simulink model "modelGreenHydrogenPlant"  (R2025a)
settings: Solver=ode1  StartTime=0.0  StopTime=exe.tsim  FixedStep=exe.tstep  RelTol=1e-3
undefined symbols (not defined in the file): Chosen_Strategy, DiscIntNeverNeededParam, ELY, ESS, exe, fb, Grid, grid, Ib2, Kc, kd, Ki_cc_cp, Ki_Inertia_Less, Kp_cc_cp, kp_GFo, Kp_Inertia_Less, PV, R, Rload, Sb, SCLR, t_ELY_on, Theta_Vvsc0, Time_Step, Va0, Vb0, Vb1, Vb2, Vc0, Vm0, VSC01_id0, Vvsc0, wb, Zb
libraries: spsSeriesRLCBranchLib x18, spsCurrentMeasurementLib x17, spsVoltageMeasurementLib x15, Control_Lib x13, spsRMSLib x8, simulink x8, spsabctodq0Lib x7, spsThreePhaseBreakerLib x5, spsPowerdq0InstantaneousLib x4, spsGroundLib x3, spsUniversalBridgeLib x3, spsControlledVoltageSourceLib x3
(part 1 of 3)
settings Model: Creator=kauchr  LastModifiedBy=kauchr
settings OptimizationCC: ReuseModelBlockBuffer=off
settings RTWCC: GPUComputeCapability=3.5

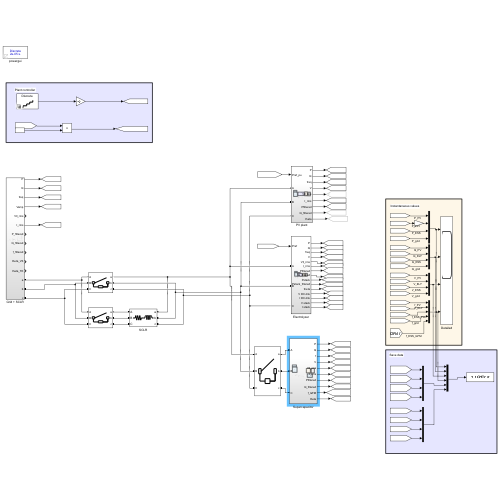
[thumbnail: Simulink's stored preview of the top-level diagram]
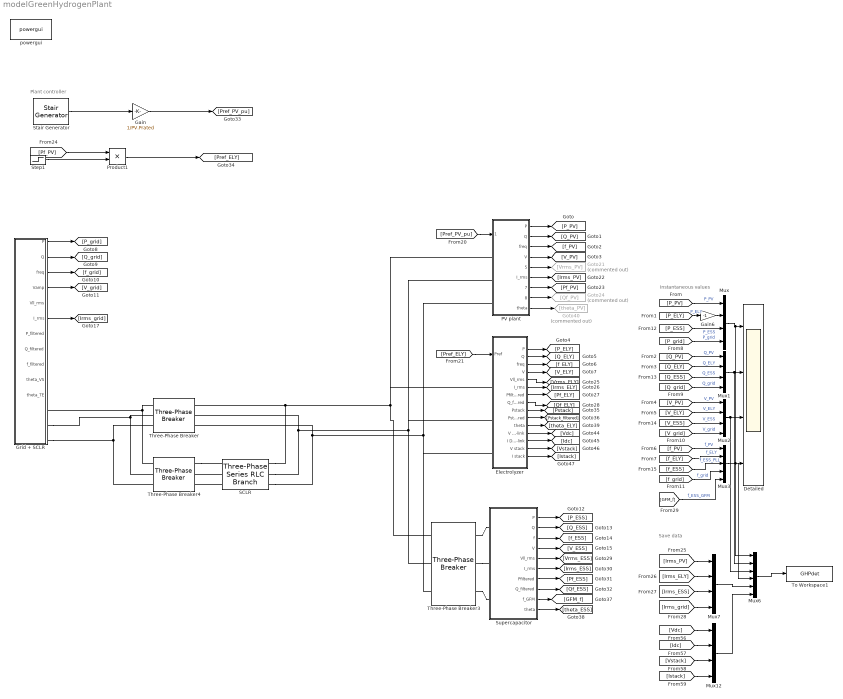
== system modelGreenHydrogenPlant ==
  note: Plant controller
  note: Instantaneous values
  note: Save data
  Detailed : Scope  NumInputPorts=4
      settings: Title=Active power  ActiveDisplayYMinimum=-22041.76945  ActiveDisplayYMaximum=60401.48573  YLabel=Active power (W)
  Electrolyzer : Subsystem
  Gain : Gain  Gain=1/PV.Prated
  Gain6 : Gain  Gain=-1
  Goto21 : Goto  Commented=on  GotoTag=Vrms_PV
  Goto24 : Goto  Commented=on  GotoTag=Qf_PV
  Goto40 : Goto  Commented=on  GotoTag=theta_PV
  Grid + SCLR : Subsystem
  Mux{,1..2,7,12} (5 alike) : Mux
  Mux3 : Mux  Inputs=5
  Mux6 : Mux  Inputs=6
  PV plant : Subsystem
  Product1 : Product
  SCLR : spsThreePhaseSeriesRLCBranchLib/Three-Phase Series RLC Branch  LConnTagsString=A|B|C  RConnTagsString=A|B|C  BranchType=RL  Resistance=SCLR.R  Inductance=SCLR.L  Capacitance=1e-6  Measurements=None
  Stair Generator : eeStairGenerator/Stair Generator  LabelModeActiveChoice=Discrete  TimeInput=setP_t  AmplitudeInput=setP_P  SampleTime=exe.tstep  RepeatPattern=off  OutDataTypeStr=double
      settings: LibrarySourceBlock=ee_sl_lib/General Control/Stair Generator
  Step1 : Step  Time=t_ELY_on  SampleTime=0
  Supercapacitor : Subsystem
  Three-Phase Breaker : spsThreePhaseBreakerLib/Three-Phase Breaker  InitialState=open  SwitchA=on  SwitchB=on  SwitchC=on  SwitchTimes="[Grid.CB.on  Grid.CB.off]"  External=off  BreakerResistance=0.01  SnubberResistance=1e6  SnubberCapacitance=inf  Measurements=None
  Three-Phase Breaker3 : spsThreePhaseBreakerLib/Three-Phase Breaker  InitialState=open  SwitchA=on  SwitchB=on  SwitchC=on  SwitchTimes="[ESS.CB.on  ESS.CB.off]"  External=off  BreakerResistance=1e-6  SnubberResistance=1e6  SnubberCapacitance=inf  Measurements=None
  Three-Phase Breaker4 : spsThreePhaseBreakerLib/Three-Phase Breaker  InitialState=open  SwitchA=on  SwitchB=on  SwitchC=on  SwitchTimes="[SCLR.CB.on  SCLR.CB.off]"  External=off  BreakerResistance=0.01  SnubberResistance=1e6  SnubberCapacitance=inf  Measurements=None
  To Workspace1 : ToWorkspace  VariableName=GHPdet  SaveFormat=Timeseries  SampleTime=1e-3
  powergui : sps_lib/powergui  Priority=1  SimulationMode=Discrete  SampleTime=exe.tstep  frequency=60  Iterations=50  frequencyindice=0  Pbase=100e6  ErrMax=1e-4  UnitsV=kV  UnitsW=MW  buscounter=0  FunctionMessages=off  echomessages=off  EnableUseOfTLC=off  CurrentSourceSwitches=off  DisableSnubberDevices=off  DisableRonSwitches=off  DisableVfSwitches=off  DisplayEquations=off  AutomaticDiscreteSolvers=off  SolverType=Tustin/Backward Euler (TBE)  Interpol=off  ExternalGateDelay=off  methode=off  Ts=100  x0status=blocks  SPID=on  SwTol=0  HookPort=off  NonlinearTolerance=1e-4  nMaxIteration=100  ContinueOnMaxIteration=off  RestoreLinks=warning  ResistiveCurrentMeasurement=off  Frange=[0:2:500]  Ylog=off  Xlog=on  ShowGrid=off  save=off  variable=ZData  structure=0  ZoomFFT=off  StartTime=0.0  cycles=1  DisplayStyle=1  fundamental=60  FreqAxis=off  MaxFrequency=1000  frequencyindicesteady=1  RmsSteady=1  display=off
  wires:
  PV plant/1(P) -> [P_PV]
  PV plant/2(Q) -> [Q_PV]
  PV plant/3(freq) -> [f_PV]
  PV plant/4(V) -> [V_PV]
  Electrolyzer/4(V) -> [V_ELY]
  Electrolyzer/1(P) -> [P_ELY]
  Electrolyzer/2(Q) -> [Q_ELY]
  Electrolyzer/3(freq) -> [f_ELY]
  [P_PV] -> Mux/1  "P_PV"
  [P_ELY] -> Gain6/1  "P_ELY"
  [Q_ELY] -> Mux1/2  "Q_ELY"
  [Q_PV] -> Mux1/1  "Q_PV"
  [V_PV] -> Mux2/1  "V_PV"
  [V_ELY] -> Mux2/2  "V_ELY"
  [f_ELY] -> Mux3/2  "f_ELY"
  [f_PV] -> Mux3/1  "f_PV"
  Mux/1 -> Mux6/1, Detailed/1
  Mux1/1 -> Mux6/2, Detailed/2
  Mux2/1 -> Mux6/3, Detailed/3
  Mux3/1 -> Mux6/4, Detailed/4
  Supercapacitor/1(P) -> [P_ESS]
  Supercapacitor/2(Q) -> [Q_ESS]
  Supercapacitor/3(f) -> [f_ESS]
  Supercapacitor/4(V) -> [V_ESS]
  [P_ESS] -> Mux/3  "P_ESS"
  [P_grid] -> Mux/4  "P_grid"
  [Q_ESS] -> Mux1/3  "Q_ESS"
  [Q_grid] -> Mux1/4  "Q_grid"
  [V_grid] -> Mux2/4  "V_grid"
  [V_ESS] -> Mux2/3  "V_ESS"
  [f_ESS] -> Mux3/3  "f_ESS_PLL"
  [f_grid] -> Mux3/4  "f_grid"
  PV plant/6(I_rms) -> [Irms_PV]
  PV plant/5(Vll_rms) -> Goto21/1
  PV plant/7(Pfiltered) -> [Pf_PV]
  PV plant/8(Q_filtered) -> Goto24/1
  Electrolyzer/5(Vll_rms) -> [Vrms_ELY]
  Electrolyzer/6(I_rms) -> [Irms_ELY]
  Electrolyzer/7(Pfiltered) -> [Pf_ELY]
  Electrolyzer/8(Q_filtered) -> [Qf_ELY]
  Supercapacitor/5(Vll_rms) -> [Vrms_ESS]
  Supercapacitor/6(I_rms) -> [Irms_ESS]
  Supercapacitor/7(Pfiltered) -> [Pf_ESS]
  Supercapacitor/8(Q_filtered) -> [Qf_ESS]
  Grid + SCLR/1(P) -> [P_grid]
  Grid + SCLR/2(Q) -> [Q_grid]
  Grid + SCLR/3(freq) -> [f_grid]
  Grid + SCLR/4(Vamp) -> [V_grid]
  Grid + SCLR/6(I_rms) -> [Irms_grid]
  [Pref_PV_pu] -> PV plant/1(Pref_pu)
  [Pref_ELY] -> Electrolyzer/1(Pref)
  Gain/1 -> [Pref_PV_pu]
  Step1/1 -> Product1/2
  Stair Generator/1 -> Gain/1
  Gain6/1 -> Mux/2
  Electrolyzer/9(Pstack) -> [Pstack]
  Electrolyzer/10(Pstack_filtered) -> [Pstack_filtered]
  [Irms_grid] -> Mux7/4
  Mux7/1 -> Mux6/5
  [Irms_PV] -> Mux7/1
  [Irms_ELY] -> Mux7/2
  Mux6/1 -> To Workspace1/1
  [Irms_ESS] -> Mux7/3
  Supercapacitor/9(f_GFM) -> [GFM_f]
  [GFM_f] -> Mux3/5  "f_ESS_GFM"
  Supercapacitor/10(theta) -> [theta_ESS]
  Electrolyzer/11(theta) -> [theta_ELY]
  PV plant/9(theta) -> Goto40/1
  [Pf_PV] -> Product1/1
  Electrolyzer/12(V DC-link) -> [Vdc]
  Electrolyzer/13(I DC-link) -> [Idc]
  Electrolyzer/14(V stack) -> [Vstack]
  Electrolyzer/15(I stack) -> [Istack]
  Mux12/1 -> Mux6/6
  [Vdc] -> Mux12/1
  [Idc] -> Mux12/2
  [Vstack] -> Mux12/3
  [Istack] -> Mux12/4
  Product1/1 -> [Pref_ELY]
  connections:
  Three-Phase Breaker/LConn1 -- Three-Phase Breaker4/LConn1 -- Grid + SCLR/RConn1
  Grid + SCLR/RConn2 -- Three-Phase Breaker/LConn2 -- Three-Phase Breaker4/LConn2
  Grid + SCLR/RConn3 -- Three-Phase Breaker/LConn3 -- Three-Phase Breaker4/LConn3
  Three-Phase Breaker4/RConn1 -- SCLR/LConn1
  SCLR/LConn3 -- Three-Phase Breaker4/RConn3
  SCLR/LConn2 -- Three-Phase Breaker4/RConn2
  Three-Phase Breaker3/RConn1 -- Supercapacitor/LConn1
  Three-Phase Breaker3/RConn2 -- Supercapacitor/LConn2
  Three-Phase Breaker3/RConn3 -- Supercapacitor/LConn3
  SCLR/RConn3 -- Three-Phase Breaker3/LConn3 -- Electrolyzer/LConn3 -- PV plant/LConn3 -- Three-Phase Breaker/RConn3
  SCLR/RConn2 -- Three-Phase Breaker/RConn2 -- Three-Phase Breaker3/LConn2 -- PV plant/LConn2 -- Electrolyzer/LConn2
  Three-Phase Breaker3/LConn1 -- PV plant/LConn1 -- Electrolyzer/LConn1 -- SCLR/RConn1 -- Three-Phase Breaker/RConn1

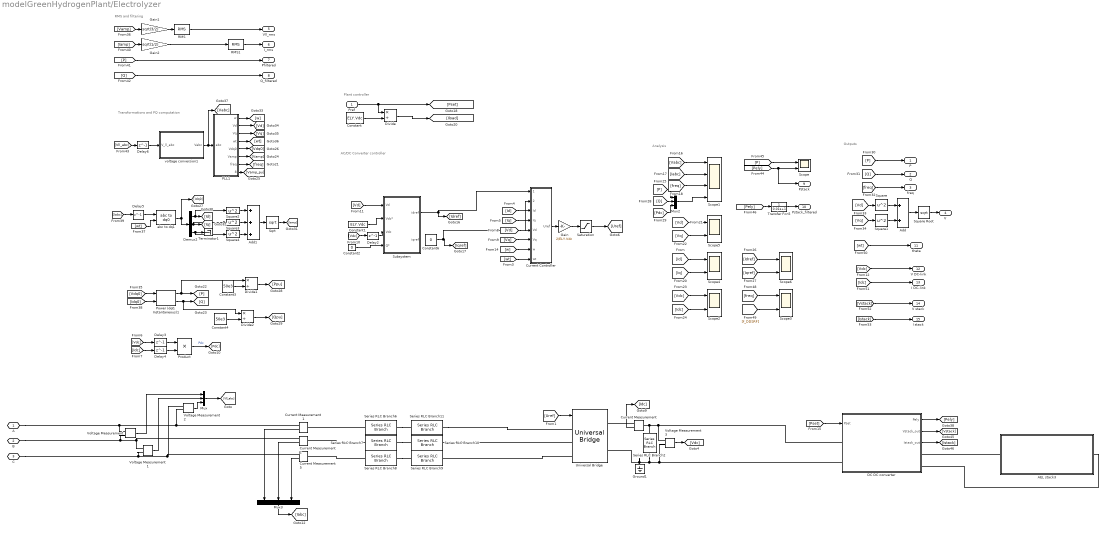
== system modelGreenHydrogenPlant/Electrolyzer ==
  note: Outputs
  note: Plant controller
  note: AC/DC Converter controller
  note: Analysis
  note: RMS and filtering
  note: Transformations and PQ computation
  Pref : Inport
  AEL stack3 : Subsystem  mask{I0_a=1650, I0_c=1650, V0_a_cell=0.25, V0_c_cell=0.25, A_cell=2000, N_cell=90, P_min_share=10, P_max_share=100, i_nom=0.165, ResultPIV=|, R_cell_ohm=0.89, Ca=1, Cc=100, a=0.04, c=0.12, i0=1.2e-4, V_rev=1.26}
      mask ResultPIV=|
      | Nominal power in kW: 56.70
      | Operating power range in kW: 5.67 - 56.70
      |
      | Nominal voltage in V: 171.81
      | Nominal current in A: 330.00
      mask prompts: I0_a "Initial resistor current at anode in A"; I0_c "Initial resistor current at cathode in A"; V0_a_cell "Initial capacitor anode cell voltage in V"; V0_c_cell "Initial capacitor cathode cell voltage in V"; A_cell "Cell active area A_cell in cm^2"; N_cell "Number of cells N_cell"; P_min_share "Minimum power in %"; P_max_share "Maximum power in %"; i_nom "Nominal current desnity in A/cm^2"; R_cell_ohm "Ohmic cell resistance in Ohm/cm^2"; Ca "Anode cell capacity in mF/cm^2"; Cc "Cathode cell capacity in mF/cm^2"; a "Anode tafel slope in V/dec"; c "Cathode tafel slope in V/dec"; i0 "Exchange current density in A/cm^2"; V_rev "Reversible cell voltage in V"
      mask DialogControl DescTextVar Prompt: Alkaline electrolyzer
      mask DialogControl Control4 Prompt: The generic alkaline electrolyzer model is based on an equivalent circuit model structure. The cathode and anode resistant are dependent on the current, wherefore initial conditions are required. Initial voltage values are needed for the constant capacitors. When connecting a current source to the electrolyzer model, the direction needs to be considered as marked. The calculated operation range does not limit the current input and is for information display only.
      mask DialogControl Container5 Prompt: References
      mask DialogControl Control5 Prompt: For more information About the model structure, see the AGISTIN Deliverable D3.2. The default parameters are taken from Sanchez-Ruiz and de Groot (https://doi.org/10.1016/j.ijhydene.2024.11.372).
      mask DialogControl Control3 Prompt: Copyright © by Fraunhofer IWES
      mask DialogControl PIV_calc Prompt: Get: power / voltage / current
      mask DialogControl PIV_calc Tooltip: Press button for calculation
      mask DialogControl Container3 Prompt: Model parameters
      mask DialogControl Container4 Prompt: Initial conditions
      mask Display: image('Mask_pic.png');
  Add : Sum
  Add1 : Sum  Inputs=+++
  Constant : Constant  Value=ELY.Vdc
  Constant1 : Constant  Value=ELY.Vdc
  Constant2 : Constant  Value=0
  Constant3 : Constant  Value=50e3
  Constant4 : Constant  Value=50e3
  Constant6 : Constant  Value=0
  "Current Controller " : Subsystem
  Current Measurement{,1..2,5} (4 alike) : spsCurrentMeasurementLib/Current Measurement  PhasorSimulation=off  OutputType=Complex  PSBequivalent=0
  DC DC converter : Subsystem
  Delay2 : Delay  DelayLength=1  InitialCondition=ELY.Vdc
  Delay3 : Delay  DelayLength=1  InitialCondition=ELY.Vdc
  Delay4 : Delay  DelayLength=1
  Delay5 : Delay  DelayLength=1
  Delay6 : Delay  DelayLength=1  InitialCondition=[489.4 0 -489.4]
  Demux2 : Demux  Outputs=3
  Divide : Product  Inputs=*/
  Divide1 : Product  Inputs=*/
  Divide2 : Product  Inputs=*/
  Gain : Gain  Gain=2/ELY.Vdc
  Gain1 : Gain  Gain=sqrt(3/2)
  Gain2 : Gain  Gain=sqrt(1/2)
  Ground1 : spsGroundLib/Ground  LConnTagsString=a
  Mux : Mux  Inputs=3
  Mux2 : Mux  Inputs=3
  Mux3 : Mux  Inputs=3
  PLL1 : Subsystem
  "Power (dq0, Instantaneous)1" : spsPowerdq0InstantaneousLib/Power (dq0, Instantaneous)
      settings: LibrarySourceBlock=|
      | sps_lib/Sensors and Measurements/Power
      | (dq0, Instantaneous)
  Product : Product
  RMS : spsRMSLib/RMS  TrueRMS=on  Freq=50  RMSInit=400  Ts=0
  RMS1 : spsRMSLib/RMS  TrueRMS=on  Freq=50  RMSInit=400  Ts=0
  Saturation : Saturate  UpperLimit=1  LowerLimit=-1
  Scope{,2..6} (6 alike) : Scope  NumInputPorts=2
      Scope settings: ActiveDisplayYMinimum=-70055.6599816338  ActiveDisplayYMaximum=113276.34782219518  DataLoggingVariableName=ScopeData2
      Scope2 settings: Title=DC-link voltage  ActiveDisplayYMinimum=90.091525350913216  ActiveDisplayYMaximum=117.90153335779667  DataLoggingVariableName=ScopeData6
      Scope3 settings: ActiveDisplayYMinimum=-2605.43865  ActiveDisplayYMaximum=6114.71016  DataLoggingVariableName=ScopeData3
      Scope4 settings: ActiveDisplayYMinimum=-132.95137  ActiveDisplayYMaximum=68.4706  DataLoggingVariableName=ScopeData4
      Scope5 settings: ActiveDisplayYMinimum=-172.28017  ActiveDisplayYMaximum=413.52414  DataLoggingVariableName=ScopeData5
      Scope6 settings: ActiveDisplayYMinimum=-2.644601079454E+7  ActiveDisplayYMaximum=2.93936985987E+6  DataLoggingVariableName=ScopeData7
  Scope1 : Scope  NumInputPorts=4
      settings: ActiveDisplayYMinimum=-430.41159  ActiveDisplayYMaximum=424.46195  DataLoggingVariableName=ScopeData3
  Series RLC Branch10 : spsSeriesRLCBranchLib/Series RLC Branch  LConnTagsString=__new0  RConnTagsString=__new0  BranchType=R  Resistance=ELY.Rc  Inductance=1e-3  SetiL0=off  InitialCurrent=0  Capacitance=1e-6  Setx0=off  InitialVoltage=0  Measurements=None
  Series RLC Branch11 : spsSeriesRLCBranchLib/Series RLC Branch  LConnTagsString=__new0  RConnTagsString=__new0  BranchType=R  Resistance=ELY.Rc  Inductance=1e-3  SetiL0=off  InitialCurrent=0  Capacitance=1e-6  Setx0=off  InitialVoltage=0  Measurements=None
  Series RLC Branch2 : spsSeriesRLCBranchLib/Series RLC Branch  LConnTagsString=__new0  RConnTagsString=__new0  BranchType=C  Resistance=Rload  Inductance=ELY.Lc  SetiL0=off  InitialCurrent=0  Capacitance=ELY.Cdc.param  Setx0=on  InitialVoltage=ELY.Vdc  Measurements=None
  Series RLC Branch6 : spsSeriesRLCBranchLib/Series RLC Branch  LConnTagsString=__new0  RConnTagsString=__new0  BranchType=L  Resistance=Rload  Inductance=ELY.Lc  SetiL0=off  InitialCurrent=0  Capacitance=1e-6  Setx0=off  InitialVoltage=0  Measurements=None
  Series RLC Branch7 : spsSeriesRLCBranchLib/Series RLC Branch  LConnTagsString=__new0  RConnTagsString=__new0  BranchType=L  Resistance=Rload  Inductance=ELY.Lc  SetiL0=off  InitialCurrent=0  Capacitance=1e-6  Setx0=off  InitialVoltage=0  Measurements=None
  Series RLC Branch8 : spsSeriesRLCBranchLib/Series RLC Branch  LConnTagsString=__new0  RConnTagsString=__new0  BranchType=L  Resistance=Rload  Inductance=ELY.Lc  SetiL0=off  InitialCurrent=0  Capacitance=1e-6  Setx0=off  InitialVoltage=0  Measurements=None
  Series RLC Branch9 : spsSeriesRLCBranchLib/Series RLC Branch  LConnTagsString=__new0  RConnTagsString=__new0  BranchType=R  Resistance=ELY.Rc  Inductance=1e-3  SetiL0=off  InitialCurrent=0  Capacitance=1e-6  Setx0=off  InitialVoltage=0  Measurements=None
  Sqrt : Sqrt
  Square{,1..4} (5 alike) : Math  Operator=square
  Square Root : Sqrt
  Subsystem : Subsystem
  Terminator1 : Terminator
  Transfer Fcn5 : TransferFcn  Denominator=[0.01 1]
  Universal Bridge : spsUniversalBridgeLib/Universal Bridge  Arms=3  SnubberResistance=1e5  SnubberCapacitance=inf  Device=Average-model based VSC  Ron=1e-3  Lon=0  ForwardVoltages="[  0  0  ]"  ForwardVoltage=0  GTOparameters=[ 10e-6 , 20e-6 ]  IGBTparameters=[ 1e-6 , 2e-6 ]  Measurements=None  Measurements_2=None  converterType=Rectifier
  Voltage Measurement{,1..3} (4 alike) : spsVoltageMeasurementLib/Voltage Measurement  PhasorSimulation=off  OutputType=Complex  PSBequivalent=0
  abc to dq1 : spsabctodq0Lib/abc to dq0  Alignment=90 degrees behind phase A axis
  voltage conversion1 : Subsystem
  A : PMIOPort  Side=Left
  B : PMIOPort  Port=2  Side=Left
  C : PMIOPort  Port=3  Side=Left
  P : Outport
  Q : Outport  Port=2
  freq : Outport  Port=3
  V : Outport  Port=4
  Vll_rms : Outport  Port=5
  I_rms : Outport  Port=6
  Pfiltered : Outport  Port=7
  Q_filtered : Outport  Port=8
  Pstack : Outport  Port=9
  Pstack_filtered : Outport  Port=10
  theta : Outport  Port=11
  V DC-link : Outport  Port=12
  I DC-link : Outport  Port=13
  V stack : Outport  Port=14
  I stack : Outport  Port=15
  wires:
  Voltage Measurement1/1 -> Mux/2
  Voltage Measurement/1 -> Mux/1
  Mux/1 -> [Vll_abc]
  Voltage Measurement2/1 -> Mux/3
  [Iq] -> "Current Controller "/4(Iq)
  [Id] -> "Current Controller "/3(Id)
  [Vd] -> "Current Controller "/5(Vd)
  [Vq] -> "Current Controller "/6(Vq)
  [Uref] -> Universal Bridge/1
  Gain/1 -> Saturation/1
  Voltage Measurement3/1 -> [Vdc]
  Product/1 -> [Pdc]  "Pdc"
  Constant1/1 -> Subsystem/2(Vdc*)
  [Vd] -> Subsystem/1(Vd)
  Constant2/1 -> Subsystem/4(Q*)
  [Vdc] -> Delay3/1
  Delay3/1 -> Product/1
  [Idc] -> Delay4/1
  Delay4/1 -> Product/2
  [wt] -> "Current Controller "/8(wt)
  [w] -> "Current Controller "/7(w)
  Pref/1 -> Divide/1, [Pset]
  Current Measurement/1 -> [Idc]
  "Current Controller "/1(Uref) -> Gain/1
  Saturation/1 -> [Uref]
  [Iabc] -> Scope1/2
  [Vabc] -> Scope1/1
  [freq] -> Scope1/3
  [Id] -> Scope4/1
  [Iq] -> Scope4/2
  [Vq] -> Scope5/2
  [Vd] -> Scope5/1
  [Idc] -> Scope2/2
  [Vdc] -> Scope2/1
  Mux2/1 -> Scope1/4
  Subsystem/1(idref) -> "Current Controller "/1(Idref), [Idref]
  [Idref] -> Scope6/1
  [Iqref] -> Scope6/2
  Delay2/1 -> Subsystem/3(Vdc)
  [Vdc] -> Delay2/1
  [P] -> Mux2/1
  [Q] -> Mux2/2
  [Pdc] -> Mux2/3
  [P] -> P/1
  [Q] -> Q/1
  [freq] -> freq/1
  [Vd] -> Square/1
  [Vq] -> Square1/1
  Square/1 -> Add/1
  Square1/1 -> Add/2
  Add/1 -> Square Root/1
  Square Root/1 -> V/1
  [Pset] -> DC DC converter/1(Pset)
  Current Measurement2/1 -> Mux3/2
  Mux3/1 -> [Iabc]
  Current Measurement1/1 -> Mux3/1
  Current Measurement5/1 -> Mux3/3
  Constant/1 -> Divide/2
  Divide/1 -> [Iload]
  Square3/1 -> Add1/2
  Square2/1 -> Add1/1
  [Iamp] -> Gain2/1
  Gain2/1 -> RMS1/1
  Divide1/1 -> [Ppu]
  Divide2/1 -> [Qpu]
  Constant3/1 -> Divide1/2
  PLL1/4(wt) -> [wt]
  [Idq0] -> "Power (dq0, Instantaneous)1"/2
  Square4/1 -> Add1/3
  abc to dq1/1 -> [Idq0], Demux2/1
  "Power (dq0, Instantaneous)1"/2 -> Divide2/1, [Q]
  PLL1/6(Vamp) -> [Vamp]
  RMS1/1 -> I_rms/1
  PLL1/7(freq) -> [freq]
  PLL1/5(Vdq0) -> [Vdq0]
  Demux2/1 -> Square2/1, [Id]
  voltage conversion1/1(Vabc) -> [Vabc], PLL1/1(abc)
  [wt] -> abc to dq1/2
  Sqrt/1 -> [Iamp]
  Delay6/1 -> voltage conversion1/1(V_ll_abc)
  [Vdq0] -> "Power (dq0, Instantaneous)1"/1
  PLL1/1(w) -> [w]
  "Power (dq0, Instantaneous)1"/1 -> Divide1/1, [P]
  Delay5/1 -> abc to dq1/1
  [Vll_abc] -> Delay6/1
  PLL1/2(Vd) -> [Vd]
  PLL1/3(Vq) -> [Vq]
  Demux2/3 -> Square4/1, Terminator1/1
  [Iabc] -> Delay5/1
  Add1/1 -> Sqrt/1
  PLL1/8(Vamp_pu) -> [Vamp_pu]
  Demux2/2 -> Square3/1, [Iq]
  Constant4/1 -> Divide2/2
  [P] -> Pfiltered/1
  [Q] -> Q_filtered/1
  DC DC converter/1(Pely) -> [Pely]
  [P] -> Scope/1
  [Pely] -> Pstack/1, Scope/2
  Transfer Fcn5/1 -> Pstack_filtered/1
  [Pely] -> Transfer Fcn5/1
  [f_DDSRF] -> Scope3/2
  [freq] -> Scope3/1
  Gain1/1 -> RMS/1
  [Vamp] -> Gain1/1
  RMS/1 -> Vll_rms/1
  [wt] -> theta/1
  Constant6/1 -> "Current Controller "/2(Iqref), [Iqref]
  DC DC converter/2(Vstack_out) -> [Vstack]
  DC DC converter/3(Istack_out) -> [Istack]
  [Istack] -> I stack/1
  [Vdc] -> V DC-link/1
  [Idc] -> I DC-link/1
  [Vstack] -> V stack/1
  connections:
  C/RConn1 -- Voltage Measurement1/LConn2 -- Current Measurement5/RConn1 -- Voltage Measurement2/LConn1
  Voltage Measurement3/LConn1 -- DC DC converter/LConn1 -- Series RLC Branch2/LConn1 -- Current Measurement/LConn1
  DC DC converter/LConn2 -- Series RLC Branch2/RConn1 -- Ground1/LConn1 -- Universal Bridge/RConn2 -- Voltage Measurement3/LConn2
  Universal Bridge/LConn3 -- Series RLC Branch9/LConn1
  Series RLC Branch8/LConn1 -- Series RLC Branch9/RConn1
  Series RLC Branch7/LConn1 -- Series RLC Branch10/RConn1
  Series RLC Branch6/LConn1 -- Series RLC Branch11/RConn1
  A/RConn1 -- Voltage Measurement2/LConn2 -- Current Measurement1/RConn1 -- Voltage Measurement/LConn1
  Voltage Measurement/LConn2 -- B/RConn1 -- Current Measurement2/RConn1 -- Voltage Measurement1/LConn1
  Series RLC Branch11/LConn1 -- Universal Bridge/LConn1
  Series RLC Branch10/LConn1 -- Universal Bridge/LConn2
  Current Measurement/RConn1 -- Universal Bridge/RConn1
  Series RLC Branch7/RConn1 -- Current Measurement2/LConn1
  Series RLC Branch8/RConn1 -- Current Measurement5/LConn1
  Series RLC Branch6/RConn1 -- Current Measurement1/LConn1
  AEL stack3/LConn1 -- DC DC converter/RConn1
  AEL stack3/RConn1 -- DC DC converter/RConn2

== system modelGreenHydrogenPlant/Grid + SCLR ==
  Constant : Constant  Value=50
  Constant1 : Constant
  "Grid " : Subsystem
  Grid impedance : spsThreePhaseSeriesRLCBranchLib/Three-Phase Series RLC Branch  LConnTagsString=A|B|C  RConnTagsString=A|B|C  BranchType=RL  Resistance=grid.R1  Inductance=grid.L1  Capacitance=1e-6  Measurements=None
  PCC : spsThreePhaseVIMeasurementLib/Three-Phase V-I Measurement  VoltageMeasurement=phase-to-ground  SetLabelV=off  LabelV=Vabc  Vpu=off  VpuLL=off  CurrentMeasurement=yes  SetLabelI=off  LabelI=Iabc  Ipu=off  Pbase=100e6  Vbase=500e3  OutputType=Complex  PhasorSimulation=off  PSBequivalent=0
  Subsystem : Subsystem
  Sum : Sum  Inputs=|++
  a : PMIOPort  Side=Right
  b : PMIOPort  Port=2  Side=Right
  c : PMIOPort  Port=3  Side=Right
  P : Outport
  Q : Outport  Port=2
  freq : Outport  Port=3
  Vamp : Outport  Port=4
  Vll_rms : Outport  Port=5
  I_rms : Outport  Port=6
  P_filtered : Outport  Port=7
  Q_filtered : Outport  Port=8
  f_filtered : Outport  Port=9
  theta_VS : Outport  Port=10
  theta_TE : Outport  Port=11
  wires:
  Subsystem/7(P_filtered) -> P_filtered/1
  PCC/1 -> Subsystem/1(Vabc)
  Constant/1 -> "Grid "/1(freq)
  Subsystem/4(Vamp) -> Vamp/1
  Subsystem/6(I_rms) -> I_rms/1
  PCC/2 -> Subsystem/2(Iabc)
  Subsystem/3(freq) -> freq/1
  Subsystem/1(P) -> P/1
  Subsystem/5(Vll_rms) -> Vll_rms/1
  Subsystem/2(Q) -> Q/1
  Subsystem/9(f_filtered) -> f_filtered/1
  Subsystem/8(Q_filtered) -> Q_filtered/1
  "Grid "/1(Theta) -> theta_VS/1
  Subsystem/10(theta) -> theta_TE/1
  Sum/1 -> "Grid "/2(Vstep_pu)
  Constant1/1 -> Sum/1
  connections:
  Grid impedance/LConn3 -- "Grid "/RConn3
  Grid impedance/RConn1 -- PCC/LConn1
  Grid impedance/RConn3 -- PCC/LConn3
  Grid impedance/LConn1 -- "Grid "/RConn1
  PCC/RConn3 -- c/RConn1
  PCC/RConn2 -- b/RConn1
  Grid impedance/LConn2 -- "Grid "/RConn2
  Grid impedance/RConn2 -- PCC/LConn2
  a/RConn1 -- PCC/RConn1

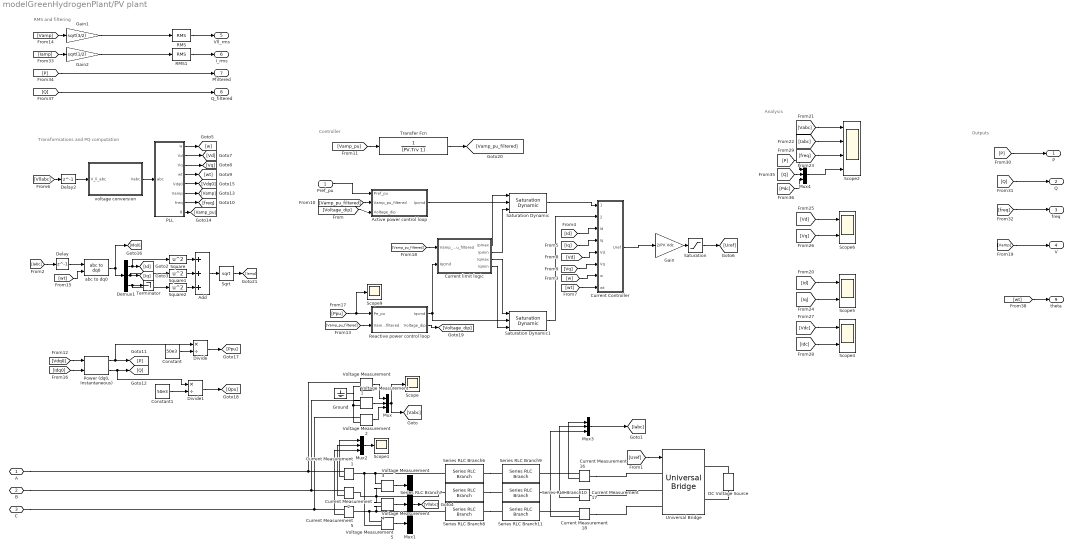
== system modelGreenHydrogenPlant/PV plant ==
  note: Controller
  note: RMS and filtering
  note: Transformations and PQ computation
  note: Analysis
  note: Outputs
  Pref_pu : Inport
  Active power control loop : Subsystem
  Add : Sum  Inputs=+++
  Constant : Constant  Value=50e3
  Constant1 : Constant  Value=50e3
  "Current Controller " : Subsystem
  Current Measurement{1..2,5,16..18} (6 alike) : spsCurrentMeasurementLib/Current Measurement  PhasorSimulation=off  OutputType=Complex  PSBequivalent=0
  Current limit logic : Subsystem
  DC Voltage Source : spsDCVoltageSourceLib/DC Voltage Source  Amplitude=PV.Vdc  Measurements=None
  Delay : Delay  DelayLength=1
  Delay2 : Delay  DelayLength=1  InitialCondition=[489.4 0 -489.4]
  Demux1 : Demux  Outputs=3
  Divide : Product  Inputs=*/
  Divide1 : Product  Inputs=*/
  Gain : Gain  Gain=2/PV.Vdc
  Gain1 : Gain  Gain=sqrt(3/2)
  Gain2 : Gain  Gain=sqrt(1/2)
  Ground : spsGroundLib/Ground  LConnTagsString=a
  Mux{,1..4} (5 alike) : Mux  Inputs=3
  PLL : Subsystem
  "Power (dq0, Instantaneous)" : spsPowerdq0InstantaneousLib/Power (dq0, Instantaneous)
      settings: LibrarySourceBlock=|
      | sps_lib/Sensors and Measurements/Power
      | (dq0, Instantaneous)
  RMS : spsRMSLib/RMS  TrueRMS=on  Freq=50  RMSInit=400  Ts=0
  RMS1 : spsRMSLib/RMS  TrueRMS=on  Freq=50  RMSInit=400  Ts=0
  Reactive power control loop : Subsystem
  Saturation : Saturate  UpperLimit=1  LowerLimit=-1
  Saturation Dynamic : simulink/Discontinuities/Saturation Dynamic  OutMin=[]  OutMax=[]  OutDataTypeStr=Inherit: Same as second input  OutDataType=fixdt(1, 16)  OutScaling=2^-10  DoSatur=off
  Saturation Dynamic1 : simulink/Discontinuities/Saturation Dynamic  OutMin=[]  OutMax=[]  OutDataTypeStr=Inherit: Same as second input  OutDataType=fixdt(1, 16)  OutScaling=2^-10  DoSatur=off
  Scope : Scope
      settings: ActiveDisplayYMinimum=-408.7778  ActiveDisplayYMaximum=408.90698
  Scope1 : Scope
      settings: ActiveDisplayYMinimum=-138.58871  ActiveDisplayYMaximum=138.55179
  Scope2 : Scope  NumInputPorts=4
      settings: ActiveDisplayYMinimum=-408.37592  ActiveDisplayYMaximum=408.37592
  Scope4 : Scope  NumInputPorts=2
      settings: ActiveDisplayYMinimum=770.40008  ActiveDisplayYMaximum=781.07031  DataLoggingVariableName=ScopeData2
  Scope5 : Scope  NumInputPorts=2
      settings: ActiveDisplayYMinimum=-13.98152  ActiveDisplayYMaximum=115.21669  DataLoggingVariableName=ScopeData3
  Scope6 : Scope  NumInputPorts=2
      settings: ActiveDisplayYMinimum=-157.63285  ActiveDisplayYMaximum=380.57215  DataLoggingVariableName=ScopeData4
  Scope9 : Scope
      settings: ActiveDisplayYMinimum=-0.13676  ActiveDisplayYMaximum=1.12677  DataLoggingVariableName=ScopeData8
  Series RLC Branch10 : spsSeriesRLCBranchLib/Series RLC Branch  LConnTagsString=__new0  RConnTagsString=__new0  BranchType=R  Resistance=PV.Rc  Inductance=1e-3  SetiL0=off  InitialCurrent=0  Capacitance=1e-6  Setx0=off  InitialVoltage=0  Measurements=None
  Series RLC Branch11 : spsSeriesRLCBranchLib/Series RLC Branch  LConnTagsString=__new0  RConnTagsString=__new0  BranchType=R  Resistance=PV.Rc  Inductance=1e-3  SetiL0=off  InitialCurrent=0  Capacitance=1e-6  Setx0=off  InitialVoltage=0  Measurements=None
  Series RLC Branch6 : spsSeriesRLCBranchLib/Series RLC Branch  LConnTagsString=__new0  RConnTagsString=__new0  BranchType=L  Resistance=Rload  Inductance=PV.Lc  SetiL0=off  InitialCurrent=0  Capacitance=1e-6  Setx0=off  InitialVoltage=0  Measurements=None
  Series RLC Branch7 : spsSeriesRLCBranchLib/Series RLC Branch  LConnTagsString=__new0  RConnTagsString=__new0  BranchType=L  Resistance=Rload  Inductance=PV.Lc  SetiL0=off  InitialCurrent=0  Capacitance=1e-6  Setx0=off  InitialVoltage=0  Measurements=None
  Series RLC Branch8 : spsSeriesRLCBranchLib/Series RLC Branch  LConnTagsString=__new0  RConnTagsString=__new0  BranchType=L  Resistance=Rload  Inductance=PV.Lc  SetiL0=off  InitialCurrent=0  Capacitance=1e-6  Setx0=off  InitialVoltage=0  Measurements=None
  Series RLC Branch9 : spsSeriesRLCBranchLib/Series RLC Branch  LConnTagsString=__new0  RConnTagsString=__new0  BranchType=R  Resistance=PV.Rc  Inductance=1e-3  SetiL0=off  InitialCurrent=0  Capacitance=1e-6  Setx0=off  InitialVoltage=0  Measurements=None
  Sqrt : Sqrt
  Square : Math  Operator=square
  Square1 : Math  Operator=square
  Square2 : Math  Operator=square
  Terminator : Terminator
  Transfer Fcn : TransferFcn  Denominator=[PV.Trv 1]
  Universal Bridge : spsUniversalBridgeLib/Universal Bridge  Arms=3  SnubberResistance=1e5  SnubberCapacitance=inf  Device=Average-model based VSC  Ron=1e-3  Lon=0  ForwardVoltages="[  0  0  ]"  ForwardVoltage=0  GTOparameters=[ 10e-6 , 20e-6 ]  IGBTparameters=[ 1e-6 , 2e-6 ]  Measurements=None  Measurements_2=None  converterType=Rectifier
  Voltage Measurement{,1..5} (6 alike) : spsVoltageMeasurementLib/Voltage Measurement  PhasorSimulation=off  OutputType=Complex  PSBequivalent=0
  abc to dq0 : spsabctodq0Lib/abc to dq0  Alignment=90 degrees behind phase A axis
  voltage conversion : Subsystem
  A : PMIOPort  Side=Left
  B : PMIOPort  Port=2  Side=Left
  C : PMIOPort  Port=3  Side=Left
  P : Outport
  Q : Outport  Port=2
  freq : Outport  Port=3
  V : Outport  Port=4
  Vll_rms : Outport  Port=5
  I_rms : Outport  Port=6
  Pfiltered : Outport  Port=7
  Q_filtered : Outport  Port=8
  theta : Outport  Port=9
  wires:
  Demux1/2 -> Square1/1, [Iq]
  Demux1/1 -> Square/1, [Id]
  PLL/4(wt) -> [wt]
  Mux2/1 -> Scope1/1
  Demux1/3 -> Square2/1, Terminator/1
  [Iabc] -> Delay/1
  Voltage Measurement1/1 -> Mux/2
  Current Measurement2/1 -> Mux2/2
  abc to dq0/1 -> [Idq0], Demux1/1
  Current Measurement1/1 -> Mux2/1
  PLL/2(Vd) -> [Vd]
  Voltage Measurement/1 -> Mux/1
  Mux/1 -> Scope/1, [Vabc]
  Voltage Measurement2/1 -> Mux/3
  PLL/3(Vq) -> [Vq]
  [w] -> "Current Controller "/7(w)
  [Iq] -> "Current Controller "/4(Iq)
  [Id] -> "Current Controller "/3(Id)
  [Vd] -> "Current Controller "/5(Vd)
  [Vq] -> "Current Controller "/6(Vq)
  [Uref] -> Universal Bridge/1
  Gain/1 -> Saturation/1
  Saturation/1 -> [Uref]
  Current Measurement5/1 -> Mux2/3
  Voltage Measurement3/1 -> Mux1/1
  Voltage Measurement4/1 -> Mux1/2
  Voltage Measurement5/1 -> Mux1/3
  Mux1/1 -> [Vllabc]
  Delay2/1 -> voltage conversion/1(V_ll_abc)
  voltage conversion/1(Vabc) -> PLL/1(abc)
  Delay/1 -> abc to dq0/1
  "Current Controller "/1(Uref) -> Gain/1
  PLL/1(w) -> [w]
  [wt] -> "Current Controller "/8(wt)
  [Vamp_pu_filtered] -> Active power control loop/2(Vamp_pu_filtered)
  "Power (dq0, Instantaneous)"/1 -> Divide/1, [P]
  [Vdq0] -> "Power (dq0, Instantaneous)"/1
  Saturation Dynamic1/1 -> "Current Controller "/2(Iqref_pu)
  Current Measurement16/1 -> Mux3/1
  Current Measurement17/1 -> Mux3/2
  Current Measurement18/1 -> Mux3/3
  Mux3/1 -> [Iabc]
  [Vamp] -> V/1
  [P] -> P/1
  [Q] -> Q/1
  [freq] -> freq/1
  PLL/7(freq) -> [freq]
  PLL/6(Vamp) -> [Vamp]
  PLL/8(Vamp_pu) -> [Vamp_pu]
  PLL/5(Vdq0) -> [Vdq0]
  [wt] -> abc to dq0/2
  [Idq0] -> "Power (dq0, Instantaneous)"/2
  Constant/1 -> Divide/2
  Constant1/1 -> Divide1/2
  "Power (dq0, Instantaneous)"/2 -> Divide1/1, [Q]
  Divide/1 -> [Ppu]
  Divide1/1 -> [Qpu]
  [Ppu] -> Scope9/1, Reactive power control loop/1(Pe_pu)
  [Vamp_pu_filtered] -> Current limit logic/1(Vamp_pu_filtered)
  Reactive power control loop/1(Iqcmd) -> Saturation Dynamic1/2, Current limit logic/2(Iqcmd)
  Active power control loop/1(Ipcmd) -> Saturation Dynamic/2
  Current limit logic/1(Ipmax) -> Saturation Dynamic/1
  Current limit logic/2(Ipmin) -> Saturation Dynamic/3
  Current limit logic/3(Iqmax) -> Saturation Dynamic1/1
  Current limit logic/4(Iqmin) -> Saturation Dynamic1/3
  Saturation Dynamic/1 -> "Current Controller "/1(Idref_pu)
  [freq] -> Scope2/3
  [Pdc] -> Mux4/3
  [Q] -> Mux4/2
  [Id] -> Scope5/1
  [Vq] -> Scope6/2
  [Vdc] -> Scope4/1
  [Vabc] -> Scope2/1
  [Idc] -> Scope4/2
  [P] -> Mux4/1
  [Vd] -> Scope6/1
  [Iq] -> Scope5/2
  [Iabc] -> Scope2/2
  Mux4/1 -> Scope2/4
  Reactive power control loop/2(Voltage_dip) -> [Voltage_dip]
  [Voltage_dip] -> Active power control loop/3(Voltage_dip)
  [Vamp_pu] -> Transfer Fcn/1
  Transfer Fcn/1 -> [Vamp_pu_filtered]
  [Vamp_pu_filtered] -> Reactive power control loop/2(Vamp_pu_filtered)
  [Vllabc] -> Delay2/1
  RMS/1 -> Vll_rms/1
  Gain1/1 -> RMS/1
  Gain2/1 -> RMS1/1
  RMS1/1 -> I_rms/1
  [P] -> Pfiltered/1
  [Q] -> Q_filtered/1
  [Vamp] -> Gain1/1
  Square/1 -> Add/1
  Square1/1 -> Add/2
  Square2/1 -> Add/3
  Add/1 -> Sqrt/1
  Sqrt/1 -> [Iamp]
  [Iamp] -> Gain2/1
  Pref_pu/1 -> Active power control loop/1(Pref_pu)
  [wt] -> theta/1
  connections:
  Voltage Measurement2/LConn2 -- Voltage Measurement/LConn2 -- Ground/LConn1 -- Voltage Measurement1/LConn2
  Current Measurement1/RConn1 -- A/RConn1 -- Voltage Measurement/LConn1
  Voltage Measurement1/LConn1 -- Current Measurement2/RConn1 -- B/RConn1
  Current Measurement5/RConn1 -- C/RConn1 -- Voltage Measurement2/LConn1
  DC Voltage Source/RConn1 -- Universal Bridge/RConn1
  DC Voltage Source/LConn1 -- Universal Bridge/RConn2
  Series RLC Branch6/RConn1 -- Series RLC Branch9/LConn1
  Series RLC Branch7/RConn1 -- Series RLC Branch10/LConn1
  Series RLC Branch8/RConn1 -- Series RLC Branch11/LConn1
  Series RLC Branch8/LConn1 -- Voltage Measurement4/LConn2 -- Voltage Measurement5/LConn1 -- Current Measurement5/LConn1
  Series RLC Branch7/LConn1 -- Voltage Measurement4/LConn1 -- Voltage Measurement3/LConn2 -- Current Measurement2/LConn1
  Series RLC Branch6/LConn1 -- Voltage Measurement3/LConn1 -- Voltage Measurement5/LConn2 -- Current Measurement1/LConn1
  Current Measurement16/LConn1 -- Universal Bridge/LConn1
  Current Measurement16/RConn1 -- Series RLC Branch9/RConn1
  Current Measurement17/LConn1 -- Universal Bridge/LConn2
  Current Measurement17/RConn1 -- Series RLC Branch10/RConn1
  Current Measurement18/LConn1 -- Universal Bridge/LConn3
  Current Measurement18/RConn1 -- Series RLC Branch11/RConn1

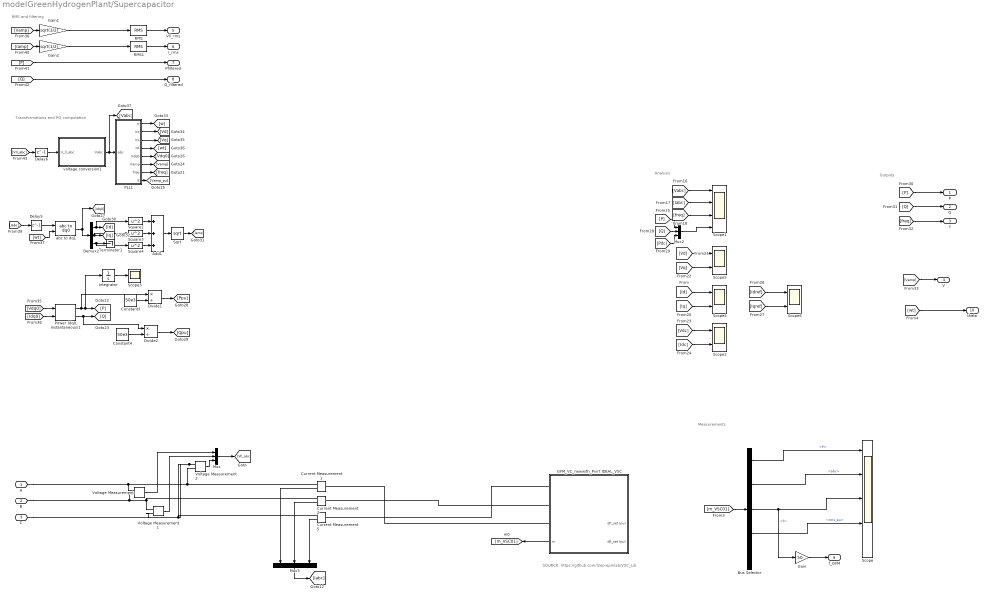
== system modelGreenHydrogenPlant/Supercapacitor ==
  note: SOURCE: https://github.com/l2ep-epmlab/VSC_Lib
  note: Analysis
  note: RMS and filtering
  note: Transformations and PQ computation
  note: Outputs
  note: Measurements
  Add1 : Sum  Inputs=+++
  Bus Selector : BusSelector  OutputSignals=P,Ig.abc,f,Ig.rms_pu,Theta
  Constant3 : Constant  Value=50e3
  Constant4 : Constant  Value=50e3
  Current Measurement1 : spsCurrentMeasurementLib/Current Measurement  PhasorSimulation=off  OutputType=Complex  PSBequivalent=0
  Current Measurement2 : spsCurrentMeasurementLib/Current Measurement  PhasorSimulation=off  OutputType=Complex  PSBequivalent=0
  Current Measurement5 : spsCurrentMeasurementLib/Current Measurement  PhasorSimulation=off  OutputType=Complex  PSBequivalent=0
  Delay5 : Delay  DelayLength=1
  Delay6 : Delay  DelayLength=1  InitialCondition=[489.4 0 -489.4]
  Demux2 : Demux  Outputs=3
  Divide1 : Product  Inputs=*/
  Divide2 : Product  Inputs=*/
  GFM_VC_newwith_Pvirt IDEAL_VSC : Subsystem  mask(VSC){fn=50, Sn=ESS.Srated, Pn=ESS.Prated, Udcn=1000, Output_Delay=100e-6, Un1=400, Un2=400, Rt_pu=0.005, Lt_pu=0.15, Lm_pu=500, Rm_pu=500, DC_Link=Perfect DC Source, H_DC=inf, H_DC_sav=inf, wn_PLL=100, zeta_PLL=1, Val_Freq_Support=off, R_percent=4, dLc_pu=0.3, Rv=0.09, W_TVR=60, I_max_pu=1.2, Tr_I_max=10, Tau_fCC=0.01, wn_CC=1200, Kffi=on, Filtre_FF=off, w_ff=1000, Advanced=on, gainpopup=With Inertia, wn_Inertia_Less=5/(2*pi), Param_Inertia=VSM, H_GFo=3, zeta_GFo=1, LFpopup=PV, P0=0.9, Q0=-0.069426, V0=1, Theta0=2.5991}
      mask prompts: fn "Nominal Frequency (Hz)"; Sn "Nominal Apparent Power (VA)"; Pn "Nominal Power (W)"; Udcn "Nominal DC Voltage (V)"; Output_Delay "Equivalent Output Delay (s)"; Un1 "VSC side Nominal Ph-Ph Voltage (V)"; Un2 "Grid side Nominal Ph-Ph Voltage (V)"; Rt_pu "R (pu)"; Lt_pu "L (pu)"; Lm_pu "Rm (pu)"; Rm_pu "Lm (pu)"; H_DC "DC inertia (ms)"; wn_PLL "Bandwidth (rad/s)"; zeta_PLL "Damping Ratio"; Val_Freq_Support "Frequency Support"; R_percent "Droop Gain (%)"; dLc_pu "Additional Virtual Impedance (pu)"; Rv "Damping Resistance (Rv)"; W_TVR "Dr filter"; I_max_pu "I max (pu)"; Tr_I_max "Current Loop time response (ms)"; Tau_fCC "Filter Time constant (s)"; wn_CC "Current Loop Bandwidth (rad/s))"; Kffi "Feedforward Enable"; Filtre_FF "Filter of ff enable"; w_ff "ff Filter Cutoff pulsation (rad/s)"; gainpopup "Strategy"; wn_Inertia_Less "Bandwidth (rad/s)"; H_GFo "Inertia H (s)"; zeta_GFo "Damping Ratio"; P0 "Initial Active Power (pu)"; Q0 "Initial Reactive Power (pu)"; V0 "Initial Voltage (pu)"; Theta0 "Initial Angle (°)"
      mask init:
      | Init_Base;
      | Init_VI;
      | Init_LF_L_modif;
      | Init_GFM_CC;
      settings: OpenFcn=|
      | NameStr = get_param(gcb,'Name');
      | open_system(gcbh, 'Mask');
      | 
      | h2AllOpenDlgs = DAStudio.ToolRoot.getOpenDialogs;
      | 
      | for i=1:length(h2AllOpenDlgs)
      |     try
      |          %disp(h2AllOpenDlgs(i).getSource.getBlock.Name);
      |         Dialog_block_name = h2AllOpenDlgs(i).getSource.getBlock.Name;
      |          %strcmp(Dialog_block_name, NameStr),
      |         if (strcmp(h2AllOpenDlgs(i).getSource.getBlock.Name, NameStr))
      |             iPos = h2AllOpenDlgs(i).position;
      |             h2AllOpenDlgs(i).position = [iPos(1)   iPos(2)   iPos(3)*1.4   iPos(4)];
      |         end
      |     end
      | end
      mask TypeOptions DC_Link: Perfect DC Source | No DC link capacitor | DC link capacitor
      mask Callback DC_Link:
      | % Get the mask parameter values. This is a cell
      | %   array of character vectors.
      | maskStr = get_param(gcb,'DC_Link');
      | p=Simulink.Mask.get(gcb);
      | 
      | % The pop-up menu is the first mask parameter.
      | %   Check the value selected in the pop-up
      | if strcmp(maskStr,'Perfect DC Source'),
      |     % Set the visibility of both parameters on when
      |     %   User-defined is selected in the pop-up.
      |     if strcmp(p.getParameter('H_DC').Visible,'on')
      |         p.getParameter('H_DC_sav').Value=p.getParameter('H_DC').Value;
      |     end
      |     p.getParameter('H_DC').Visible='off';
      |     p.getParameter('H_DC').Value='inf';
      | elseif strcmp(maskStr,'No DC link capacitor'),
      |     if strcmp(p.getParameter('H_DC').Visible,'on')
      |         p.getParameter('H_DC_sav').Value=p.getParameter('H_DC').Value;
      |     end
      |     p.getParameter('H_DC').Visible='off';
      |     p.getParameter('H_DC').Value='0';
      | else
      |     % Set the visibility of both parameters on when
      |     %   User-defined is selected in the pop-up.
      |     p.getParameter('H_DC').Visible='on';
      |     p.getParameter('H_DC').Value=p.getParameter('H_DC_sav').Value;
      | end
      mask Callback Advanced:
      | % Get the mask parameter values. This is a cell
      | %   array of character vectors.
      | maskStr = get_param(gcb,'Advanced');
      | p=Simulink.Mask.get(gcb);
      | 
      | % The pop-up menu is the first mask parameter.
      | %   Check the value selected in the pop-up
      | if strcmp(maskStr,'on'),
      | 
      |     % Set the visibility of both parameters on when
      |     %   User-defined is selected in the pop-up.
      |     %p.getDialogControl('TVR').Visible='on';
      |     %p.getDialogControl('TVI').Visible='on';
      |     %p.getDialogControl('LC_Filter').Visible='on';
      |     p.getDialogControl('Current_Sat').Visible='on';
      |     p.getDialogControl('CC').Visible='on';
      |     %p.getDialogControl('Param_Strat_3').Visible='off';
      | 
      | 
      | else
      | 
      |     % Set the visibility of both parameters on when
      |     %   User-defined is selected in the pop-up.
      |     %p.getDialogControl('TVR').Visible='off';
      |     %p.getDialogControl('TVI').Visible='off';
      |     %p.getDialogControl('LC_Filter').Visible='off';
      |     p.getDialogControl('Current_Sat').Visible='off';
      |     p.getDialogControl('CC').Visible='off';
      |     %p.getDialogControl('Param_Strat_3').Visible='off';
      | 
      | end
      mask TypeOptions gainpopup: Inertia Less | With Inertia
      mask Callback gainpopup:
      | % Get the mask parameter values. This is a cell
      | %   array of character vectors.
      | maskStr = get_param(gcb,'gainpopup');
      | p=Simulink.Mask.get(gcb);
      | 
      | % The pop-up menu is the first mask parameter.
      | %   Check the value selected in the pop-up
      | if strcmp(maskStr,'Inertia Less'),
      | 
      |     % Set the visibility of both parameters on when
      |     %   User-defined is selected in the pop-up.
      |     p.getDialogControl('No_Inertia').Visible='on';
      |     p.getDialogControl('Inertia').Visible='off';
      |     %p.getDialogControl('Param_Strat_3').Visible='off';
      | 
      | 
      | elseif strcmp(maskStr,'With Inertia'),
      | 
      |     % Set the visibility of both parameters on when
      |     %   User-defined is selected in the pop-up.
      |     p.getDialogControl('No_Inertia').Visible='off';
      |     p.getDialogControl('Inertia').Visible='on';
      |     %p.getDialogControl('Param_Strat_3').Visible='off';
      | 
      | 
      |     % Turn off the visibility of the Value field
      |     %   when User-defined is not selected.
      | 
      | else
      | 
      |     % Set the visibility of both parameters on when
      |     %   User-defined is selected in the pop-up.
      |     p.getDialogControl('No_Inertia').Visible='off';
      |     p.getDialogControl('Inertia').Visible='off';
      |     %p.getDialogControl('Param_Strat_3').Visible='off';
      | 
      | end
      mask TypeOptions Param_Inertia: VSM | PI
      mask TypeOptions LFpopup: Swing | PQ | PV
      mask Callback LFpopup:
      | % Get the mask parameter values. This is a cell
      | %   array of character vectors.
      | maskStr = get_param(gcb,'LFpopup');
      | p=Simulink.Mask.get(gcb);
      | 
      | % The pop-up menu is the first mask parameter.
      | %   Check the value selected in the pop-up
      | if strcmp(maskStr,'Swing'),
      | 
      |     % Set the visibility of both parameters on when
      |     %   User-defined is selected in the pop-up.
      |     p.getParameter('P0').Visible='off';
      |     p.getParameter('Q0').Visible='off';
      |     p.getParameter('V0').Visible='on';
      |     p.getParameter('Theta0').Visible='on';
      |     set_param([gcb '/Source_For_LF'],'BusType','swing');
      | 
      | elseif strcmp(maskStr,'PQ'),
      | 
      |     % Set the visibility of both parameters on when
      |     %   User-defined is selected in the pop-up.
      |     p.getParameter('P0').Visible='on';
      |     p.getParameter('Q0').Visible='on';
      |     p.getParameter('V0').Visible='off';
      |     p.getParameter('Theta0').Visible='off';
      |     set_param([gcb '/Source_For_LF'],'BusType','PQ');
      | 
      |     % Turn off the visibility of the Value field
      |     %   when User-defined is not selected.
      | else
      | 
      |     % Set the visibility of both parameters on when
      |     %   User-defined is selected in the pop-up.
      |     p.getParameter('P0').Visible='on';
      |     p.getParameter('Q0').Visible='off';
      |     p.getParameter('V0').Visible='on';
      |     p.getParameter('Theta0').Visible='off';
      |     set_param([gcb '/Source_For_LF'],'BusType','PV');
      | 
      | end
      mask DialogControl Nominal_Param Prompt: Nominal Value
      mask DialogControl Container20 Prompt: Passive Components
      mask DialogControl Container26 Prompt: Output Transformer
      mask DialogControl Container27 Prompt: DC Link
      mask DialogControl Control_Param Prompt: Control Parameter
      mask DialogControl Container13 Prompt: PLL
      mask DialogControl Container14 Prompt: Frequency Support
      mask DialogControl VI Prompt: Virtual Impedance
      mask DialogControl TVR Prompt: Transient Virtual Resistor
      mask DialogControl Current_Sat Prompt: Current Limitation
      mask DialogControl CC Prompt: Current Loop
      mask DialogControl Container18 Prompt: Control Strategy
      mask DialogControl LF_Param Prompt: Loadflow
      mask DialogControl Control4 Prompt: Initial Operating Point
      mask DialogControl Container24 Prompt: VSC side
      mask DialogControl LF_vsc_str Prompt: V0 = 1.0552 pu, Angle = 25.2352°
      mask DialogControl Container25 Prompt: PCC
      mask DialogControl LF_pcc_str Prompt: V0 = 1 pu, Angle = 2.5991°
      mask DialogControl LF_pcc_Power_str Prompt: P0 = 0.9 pu, Q0 = -0.069426 pu
      mask DialogControl UpdateLoadflow Prompt: Update Loadflow
      mask DialogControl UpdateLoadflow Callback: LoadFlow_VSC
      mask Display:
      | x1=0.05;
      | y1=0.2;
      | %
      | plot([0.5 0.5]+x1,[0.97,0.8]-y1)
      | plot([0.5 0.32]+x1,[0.80 0.71]-y1)
      | plot([0.32 0.32]+x1,[0.80 0.52]-y1)
      | plot([0.32 0.5]+x1,[0.62 0.52]-y1)
      | plot([0.5 0.5]+x1,[0.52 0.35]-y1)
      | plot([0.45 0.5 0.43]+x1,[0.59 0.52 0.51]-y1)
      | %
      | plot([0.28 0.28]+x1,[0.74 0.58]-y1)
      | plot([0.28 0.20]+x1,[0.66 0.66]-y1)
      | %
      | plot([0.5 0.63]+x1,[0.84 0.84]-y1)
      | plot([0.63 0.63]+x1,[0.84 0.72]-y1)
      | plot([0.63 0.59]+x1,[0.72 0.65]-y1)
      | plot([0.63 0.67]+x1,[0.72 0.65]-y1)
      | plot([0.59 0.67]+x1,[0.65 0.65]-y1)
      | plot([0.63 0.63]+x1,[0.65 0.47]-y1)
      | plot([0.5 0.63]+x1,[0.47 0.47]-y1)
      | plot([0.58 0.67]+x1,[0.72 0.72]-y1)
      | %
      | color('blue')
      | text(0.3,0.10,'L-Filter GFM CC')
      | 
      | port_label('input',1,'\DeltaE (pu)','texmode','on');
      | port_label('input',2,'\DeltaP (pu)','texmode','on');
      | port_label('output',1,'m');
      | port_label('rconn',1,'A');
      | port_label('rconn',2,'B');
      | port_label('rconn',3,'C');
      | port_label('lconn',1,'+');
      | port_label('lconn',2,'-');
  Gain : Gain  Gain=50
  Gain1 : Gain  Gain=sqrt(3/2)
  Gain2 : Gain  Gain=sqrt(1/2)
  Integrator : Integrator
  Mux : Mux  Inputs=3
  Mux2 : Mux  Inputs=3
  Mux3 : Mux  Inputs=3
  PLL1 : Subsystem
  "Power (dq0, Instantaneous)1" : spsPowerdq0InstantaneousLib/Power (dq0, Instantaneous)
      settings: LibrarySourceBlock=|
      | sps_lib/Sensors and Measurements/Power
      | (dq0, Instantaneous)
  RMS : spsRMSLib/RMS  TrueRMS=on  Freq=50  RMSInit=400  Ts=0
  RMS1 : spsRMSLib/RMS  TrueRMS=on  Freq=50  RMSInit=400  Ts=0
  Scope : Scope  NumInputPorts=5
      settings: ActiveDisplayYMinimum=-11.7999  ActiveDisplayYMaximum=2.34338  DataLoggingVariableName=ScopeData5
  Scope1 : Scope  NumInputPorts=4
      settings: ActiveDisplayYMinimum=-408.25999  ActiveDisplayYMaximum=408.25111  DataLoggingVariableName=ScopeData2
  Scope{2,4..6} (4 alike) : Scope  NumInputPorts=2
      Scope2 settings: ActiveDisplayYMinimum=770.40008  ActiveDisplayYMaximum=781.07031  DataLoggingVariableName=ScopeData3
      Scope4 settings: ActiveDisplayYMinimum=-31.96578  ActiveDisplayYMaximum=24.72092  DataLoggingVariableName=ScopeData4
      Scope5 settings: ActiveDisplayYMinimum=-236.96822  ActiveDisplayYMaximum=486.73389  DataLoggingVariableName=ScopeData5
      Scope6 settings: ActiveDisplayYMinimum=-216.4277  ActiveDisplayYMaximum=24.04752  DataLoggingVariableName=ScopeData6
  Scope3 : Scope
      settings: ActiveDisplayYMinimum=-0.93484  ActiveDisplayYMaximum=8.41353  DataLoggingVariableName=ScopeData2
  Sqrt : Sqrt
  Square2 : Math  Operator=square
  Square3 : Math  Operator=square
  Square4 : Math  Operator=square
  Terminator1 : Terminator
  Voltage Measurement : spsVoltageMeasurementLib/Voltage Measurement  PhasorSimulation=off  OutputType=Complex  PSBequivalent=0
  Voltage Measurement1 : spsVoltageMeasurementLib/Voltage Measurement  PhasorSimulation=off  OutputType=Complex  PSBequivalent=0
  Voltage Measurement2 : spsVoltageMeasurementLib/Voltage Measurement  PhasorSimulation=off  OutputType=Complex  PSBequivalent=0
  abc to dq1 : spsabctodq0Lib/abc to dq0  Alignment=90 degrees behind phase A axis
  voltage conversion1 : Subsystem
  A : PMIOPort  Side=Left
  B : PMIOPort  Port=2  Side=Left
  C : PMIOPort  Port=3  Side=Left
  P : Outport
  Q : Outport  Port=2
  f : Outport  Port=3
  V : Outport  Port=4
  Vll_rms : Outport  Port=5
  I_rms : Outport  Port=6
  Pfiltered : Outport  Port=7
  Q_filtered : Outport  Port=8
  f_GFM : Outport  Port=9
  theta : Outport  Port=10
  wires:
  [Vabc] -> Scope1/1
  [P] -> Mux2/1
  [Idref] -> Scope6/1
  [Iqref] -> Scope6/2
  [Iabc] -> Scope1/2
  Mux2/1 -> Scope1/4
  [Iq] -> Scope4/2
  [Q] -> Mux2/2
  [Vq] -> Scope5/2
  [Vd] -> Scope5/1
  [freq] -> Scope1/3
  [Vdc] -> Scope2/1
  [Id] -> Scope4/1
  [Idc] -> Scope2/2
  [Pdc] -> Mux2/3
  Current Measurement5/1 -> Mux3/3
  Current Measurement1/1 -> Mux3/1
  Mux3/1 -> [Iabc]
  Mux/1 -> [Vll_abc]
  Voltage Measurement2/1 -> Mux/3
  Current Measurement2/1 -> Mux3/2
  Voltage Measurement1/1 -> Mux/2
  Voltage Measurement/1 -> Mux/1
  Delay6/1 -> voltage conversion1/1(V_ll_abc)
  [wt] -> abc to dq1/2
  PLL1/1(w) -> [w]
  [Vdq0] -> "Power (dq0, Instantaneous)1"/1
  Sqrt/1 -> [Iamp]
  PLL1/5(Vdq0) -> [Vdq0]
  PLL1/7(freq) -> [freq]
  [Vamp] -> Gain1/1
  PLL1/6(Vamp) -> [Vamp]
  "Power (dq0, Instantaneous)1"/2 -> Divide2/1, [Q]
  abc to dq1/1 -> [Idq0], Demux2/1
  Demux2/1 -> Square2/1, [Id]
  RMS1/1 -> I_rms/1
  Square4/1 -> Add1/3
  Constant3/1 -> Divide1/2
  [Idq0] -> "Power (dq0, Instantaneous)1"/2
  PLL1/4(wt) -> [wt]
  [Q] -> Q_filtered/1
  Square2/1 -> Add1/1
  voltage conversion1/1(Vabc) -> [Vabc], PLL1/1(abc)
  Square3/1 -> Add1/2
  [Iamp] -> Gain2/1
  RMS/1 -> Vll_rms/1
  Demux2/2 -> Square3/1, [Iq]
  Add1/1 -> Sqrt/1
  Gain1/1 -> RMS/1
  PLL1/8(Vamp_pu) -> [Vamp_pu]
  Divide2/1 -> [Qpu]
  PLL1/3(Vq) -> [Vq]
  [P] -> Pfiltered/1
  [Vll_abc] -> Delay6/1
  Divide1/1 -> [Ppu]
  "Power (dq0, Instantaneous)1"/1 -> Divide1/1, Integrator/1, [P]
  Demux2/3 -> Square4/1, Terminator1/1
  Delay5/1 -> abc to dq1/1
  Gain2/1 -> RMS1/1
  PLL1/2(Vd) -> [Vd]
  Constant4/1 -> Divide2/2
  [Iabc] -> Delay5/1
  [Vamp] -> V/1
  [P] -> P/1
  [Q] -> Q/1
  [freq] -> f/1
  GFM_VC_newwith_Pvirt IDEAL_VSC/1(m) -> [m_VSC01]
  Bus Selector/3 -> Gain/1, Scope/3  "<f>"
  [m_VSC01] -> Bus Selector/1
  Bus Selector/1 -> Scope/1  "<P>"
  Bus Selector/2 -> Scope/2  "<abc>"
  Bus Selector/4 -> Scope/4  "<rms_pu>"
  Gain/1 -> f_GFM/1
  [wt] -> theta/1
  Integrator/1 -> Scope3/1
  connections:
  Voltage Measurement/LConn2 -- B/RConn1 -- Current Measurement2/RConn1 -- Voltage Measurement1/LConn1
  Voltage Measurement2/LConn1 -- C/RConn1 -- Voltage Measurement1/LConn2 -- Current Measurement5/RConn1
  Current Measurement1/RConn1 -- A/RConn1 -- Voltage Measurement/LConn1 -- Voltage Measurement2/LConn2
  GFM_VC_newwith_Pvirt IDEAL_VSC/RConn1 -- Current Measurement1/LConn1
  GFM_VC_newwith_Pvirt IDEAL_VSC/RConn2 -- Current Measurement2/LConn1
  GFM_VC_newwith_Pvirt IDEAL_VSC/RConn3 -- Current Measurement5/LConn1
